simulink model "lab04z3_sch"  (Simulink 10.3)
settings: Solver=VariableStepAuto  StartTime=0.0  StopTime=10  FixedStep=0.001  MaxStep=0.001  RelTol=1e-3  EnableMultiTasking=on
InitFcn:
  | % Parametry obiektu
  | R = 3;
  | L = 0.05;
  | kfi = 2.23;
  | J = 0.11;
  | % Okres probkowania
values from neighbouring files (symbols this model uses):
  ki = 1    [lab04z1.m]
  Kx = acker(A, B, [-wc, -wc])    [lab04z1.m]
undefined symbols (not defined in the file or in its folder): regStan, Tp
settings Model: Creator=Jacek  LastModifiedBy=AgraWoodAdmin
settings DataIOCC: LimitDataPoints=on  SignalLoggingSaveFormat=Dataset
settings OptimizationCC: ExpressionDepthLimit=128
settings DebuggingCC: UnderspecifiedInitializationDetection=Simplified  MergeDetectMultiDrivingBlocksExec=error  SolverPrmCheckMsg=warning  FcnCallInpInsideContextMsg=error  StateNameClashWarn=none
settings GRTTargetCC: CombineOutputUpdateFcns=on  GRTInterface=off
settings ConfigComp: CovSFcnEnable=off

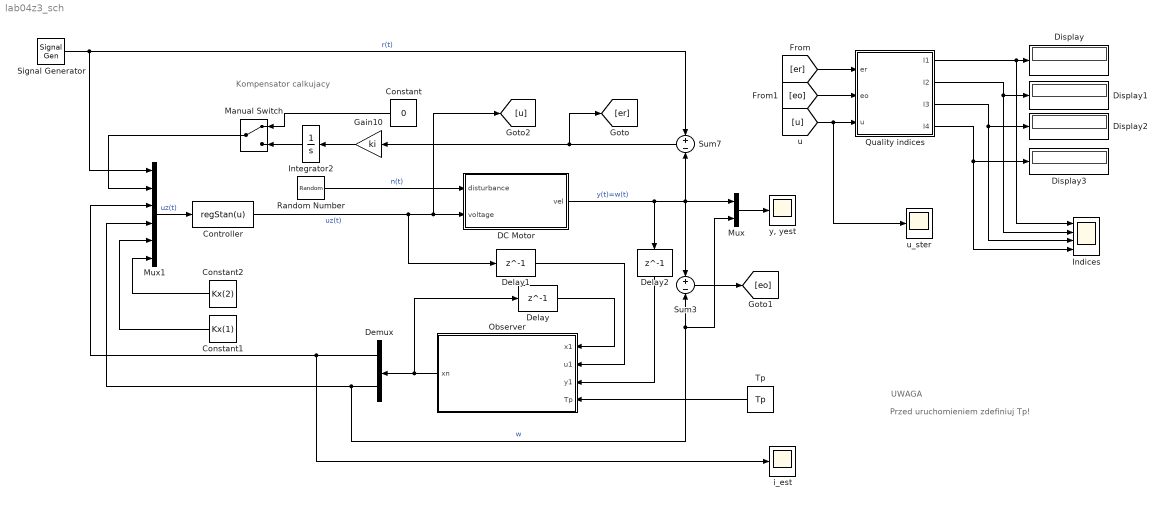
== system lab04z3_sch ==
  note: Przed uruchomieniem zdefiniuj Tp!
  note: UWAGA
  note: Kompensator calkujacy
  Constant : Constant  Value=0
  Constant1 : Constant  Value=Kx(1)
  Constant2 : Constant  Value=Kx(2)
  Controller : MATLABFcn  MATLABFcn=regStan(u)  OutputDimensions=1
  DC Motor : Subsystem
  Delay : Delay  DelayLength=1  InitialCondition=[40.0; 20.0]
  Delay1 : Delay  DelayLength=1
  Delay2 : Delay  DelayLength=1
  Demux : Demux  Outputs=2
  Display{,1..3} (4 alike) : Display
  Gain10 : Gain  Gain=ki
  Indices : Scope  NumInputPorts=4
  Integrator2 : Integrator
  Manual Switch : ManualSwitch
  Mux : Mux  Inputs=2
  Mux1 : Mux  Inputs=6
  Observer : MATLAB Function  TreatAsAtomicUnit=on
  Quality indices : Subsystem
  Random Number : RandomNumber  Variance=10
  Signal Generator : SignalGenerator  WaveForm=square  Amplitude=200  Frequency=0.5
  Sum3 : Sum  Inputs=+|-
  Sum7 : Sum  Inputs=+|-
  Tp : Constant  Value=Tp
  i_est : Scope
  u_ster : Scope
  "y, yest" : Scope
  wires:
  Random Number/1 -> DC Motor/1(disturbance)  "n(t)"
  Controller/1 -> [u], DC Motor/2(voltage), Delay1/1  "uz(t)"
  DC Motor/1(vel) -> Delay2/1, Sum3/1, Sum7/2, Mux/1  "y(t)=w(t)"
  Sum3/1 -> [eo]
  Mux/1 -> "y, yest"/1
  Signal Generator/1 -> Sum7/1, Mux1/1  "r(t)"
  Integrator2/1 -> Manual Switch/2
  Sum7/1 -> [er], Gain10/1
  Gain10/1 -> Integrator2/1
  Manual Switch/1 -> Mux1/2
  Constant/1 -> Manual Switch/1
  Quality indices/4(I4) -> Indices/4, Display3/1
  Quality indices/1(I1) -> Indices/1, Display/1
  Quality indices/2(I2) -> Display1/1, Indices/2
  Quality indices/3(I3) -> Display2/1, Indices/3
  [er] -> Quality indices/1(er)
  [eo] -> Quality indices/2(eo)
  [u] -> u_ster/1, Quality indices/3(u)
  Observer/1(xn) -> Demux/1, Delay/1
  Delay1/1 -> Observer/2(u1)
  Delay2/1 -> Observer/3(y1)
  Tp/1 -> Observer/4(Tp)
  Demux/2 -> Mux1/4, Mux/2, Sum3/2  "w"
  Delay/1 -> Observer/1(x1)
  Demux/1 -> Mux1/3, i_est/1
  Mux1/1 -> Controller/1  "uz(t)"
  Constant2/1 -> Mux1/6
  Constant1/1 -> Mux1/5

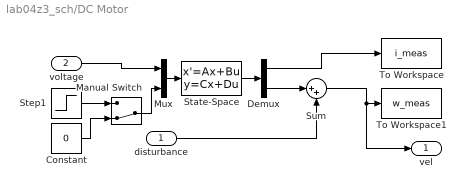
== system lab04z3_sch/DC Motor ==
  disturbance : Inport
  voltage : Inport  Port=2
  Constant : Constant  Value=0
  Demux : Demux  Outputs=2
  Manual Switch : ManualSwitch  CurrentSetting=0
  Mux : Mux  Inputs=2
  State-Space : StateSpace  A=[-3/0.05, -2.23/0.05; 2.23/0.11, 0]  B=[1/0.05 0; 0 -1/0.11]  C=[1 0;0 1]  D=[0 0; 0 0]  InitialCondition=[0 ;40]
  Step1 : Step  Time=0.5  After=44.6*1  SampleTime=0
  Sum : Sum  Inputs=|++
  To Workspace : ToWorkspace  VariableName=i_meas  SampleTime=-1
  To Workspace1 : ToWorkspace  VariableName=w_meas  SampleTime=-1
  vel : Outport  VectorParamsAs1DForOutWhenUnconnected=off
  wires:
  Mux/1 -> State-Space/1
  voltage/1 -> Mux/1
  Step1/1 -> Manual Switch/1
  State-Space/1 -> Demux/1
  Demux/1 -> To Workspace/1
  disturbance/1 -> Sum/2
  Sum/1 -> vel/1, To Workspace1/1
  Demux/2 -> Sum/1
  Manual Switch/1 -> Mux/2
  Constant/1 -> Manual Switch/2

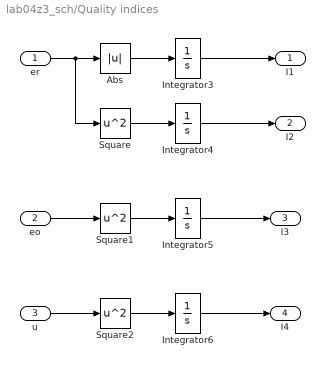
== system lab04z3_sch/Quality indices ==
  er : Inport
  eo : Inport  Port=2
  u : Inport  Port=3
  Abs : Abs
  Integrator{3..6} (4 alike) : Integrator
  Square : Math  Operator=square  SignedPower=on  RndMeth=Zero  SaturateOnIntegerOverflow=on
  Square1 : Math  Operator=square  SignedPower=on  RndMeth=Zero  SaturateOnIntegerOverflow=on
  Square2 : Math  Operator=square  SignedPower=on  RndMeth=Zero  SaturateOnIntegerOverflow=on
  I1 : Outport  VectorParamsAs1DForOutWhenUnconnected=off
  I2 : Outport  Port=2  VectorParamsAs1DForOutWhenUnconnected=off
  I3 : Outport  Port=3  VectorParamsAs1DForOutWhenUnconnected=off
  I4 : Outport  Port=4  VectorParamsAs1DForOutWhenUnconnected=off
  wires:
  eo/1 -> Square1/1
  Square2/1 -> Integrator6/1
  Integrator6/1 -> I4/1
  u/1 -> Square2/1
  er/1 -> Abs/1, Square/1
  Integrator4/1 -> I2/1
  Square1/1 -> Integrator5/1
  Integrator5/1 -> I3/1
  Abs/1 -> Integrator3/1
  Integrator3/1 -> I1/1
  Square/1 -> Integrator4/1

== matlab function Observer ==
  settings: updateMethod=DISCRETE  sampleTime=Tp
  data: x1 input double; u1 input double; y1 input double; xn output double; Tp input double
function xn  = discreteObserver(x1, u1, y1, Tp)

% Uwaga: indeks 1, bo zgodnie z (4) wszystki sygnaly opoznione o probke.

% Model i jego parametry
R = 3;      % [Om]
L = 0.05;   % [H]
kfi = 2.23; % [Vs^2]
J = 0.11;   % [Nm^2]
% Macierze rownan stanu
A = [-R/L, -kfi/L; kfi/J, 0];
B = [1/L; 0]; C = [0, 1];

% Wzmocnienia obserwatora - wyliczone wczesniej
Lo = [-44.6; 60.0];

% Obliczenie estymat
xn = (eye(2)+A*Tp)*x1 + B*Tp*u1 + Lo*Tp*(y1-C*x1);
